simulink model "torqueWalking"  (Simulink 8.9)
settings: Solver=FixedStepAuto  StartTime=0.0  StopTime=CONFIG.SIMULATION_TIME  FixedStep=CONFIG.Ts  RelTol=1e-3
InitFcn:
  | initTorqueWalking
undefined symbols (not defined in the file or in its folder): CONFIG, frictionConeConstraintsMatrix, gain, reg, ROBOT_DOF, root_displacement, upperBoundFrictionConeConstraints, WBT_robotName
undefined symbols (not defined in the file): sat
libraries: WBToolboxLibrary x35
settings Model: SuppressorTable=22 serialization::archive 11 0 6 0 0 0 11 0  Creator=mcharbonneau  LastModifiedBy=mcharbonneau
settings DataIOCC: LimitDataPoints=off  SaveFormat=Dataset  SignalLoggingSaveFormat=Dataset
settings OptimizationCC: LifeSpan=auto
settings DebuggingCC: UnderspecifiedInitializationDetection=Simplified  MergeDetectMultiDrivingBlocksExec=error  FcnCallInpInsideContextMsg=error  StateNameClashWarn=none  SFUnexpectedBacktrackingDiag=error  SFNoUnconditionalDefaultTransitionDiag=error  SFExecutionAtInitializationDiag=warning
settings HardwareCC: ProdBitPerPointer=64  ProdBitPerSizeT=64  ProdBitPerPtrDiffT=64  ProdLargestAtomicFloat=Float  ProdIntDivRoundTo=Zero  ProdEndianess=LittleEndian  ProdWordSize=64  ProdHWDeviceType=Intel->x86-64 (Windows64)
settings ModelReferenceCC: PropagateSignalLabelsOutOfModel=on
settings GRTTargetCC: TargetLangStandard=C99 (ISO)  GeneratePreprocessorConditionals=Use local settings  CombineOutputUpdateFcns=on  GRTInterface=off
settings ConfigComp: CovMetricSettings=dwe  CovHtmlReporting=off  CovSaveCumulativeToWorkspaceVar=off  CovSaveSingleToWorkspaceVar=off  CovExternalEMLEnable=on

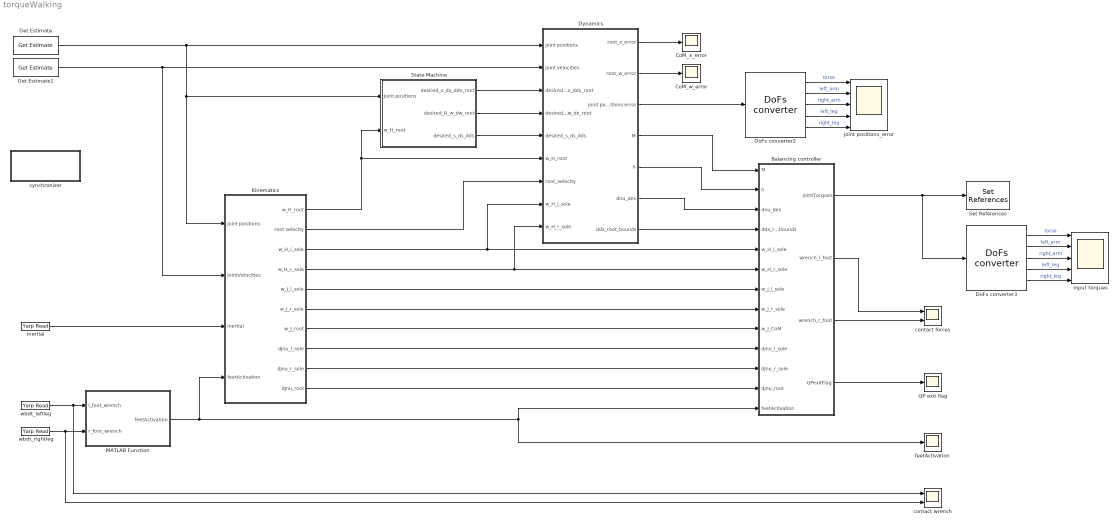
== system torqueWalking ==
  Balancing controller : Subsystem
  CoM_w_error : Scope
  CoM_x_error : Scope
  DoFs converter2 : WBToolboxLibrary/Utilities/DoFs converter  yarp2WBIOption=From WBI to YARP  robotName=WBT_robotName  localName=WBT_modelName  wbiFile=WBT_wbiFilename  wbiList=WBT_wbiList
      settings: SourceProductName=Whole Body Toolbox
  DoFs converter3 : WBToolboxLibrary/Utilities/DoFs converter  yarp2WBIOption=From WBI to YARP  robotName=WBT_robotName  localName=WBT_modelName  wbiFile=WBT_wbiFilename  wbiList=WBT_wbiList
      settings: SourceProductName=Whole Body Toolbox
  Dynamics : Subsystem
  Get Estimate : WBToolboxLibrary/wholeBodyStates/Get Estimate  estimateType=Joints Position  robotName=WBT_robotName  localName=WBT_modelName  wbiFile=WBT_wbiFilename  wbiList=WBT_wbiList
      settings: SourceProductName=Whole Body Toolbox
  Get Estimate1 : WBToolboxLibrary/wholeBodyStates/Get Estimate  estimateType=Joints Velocity  robotName=WBT_robotName  localName=WBT_modelName  wbiFile=WBT_wbiFilename  wbiList=WBT_wbiList
      settings: SourceProductName=Whole Body Toolbox
  Kinematics : Subsystem
  MATLAB Function : MATLAB Function  TreatAsAtomicUnit=on
  QP exit flag : Scope
  Set References : WBToolboxLibrary/wholeBodyActuators/Set References  controlType=Torque  fullOrSubControl=Full  controlledJoints=''  robotName=WBT_robotName  localName=WBT_modelName  wbiFile=WBT_wbiFilename  wbiList=WBT_wbiList
      settings: SourceProductName=Whole Body Toolbox
  State Machine : Subsystem
  contact forces : Scope  NumInputPorts=2
  contact wrench : Scope  NumInputPorts=2
  feetActivation : Scope
  inertial : WBToolboxLibrary/Utilities/Yarp Read  portName=PORTS.IMU  signalSize=12  blocking=off  timestamp=off  autoconnect=on  errorOnConnection=on
      settings: SourceProductName=Whole Body Toolbox
  input torques : Scope  NumInputPorts=5
  joint positions_error : Scope  NumInputPorts=5
  synchronizer : Subsystem
      mask Display: disp('SYNCHRONIZER')
  wbdt_leftleg : WBToolboxLibrary/Utilities/Yarp Read  portName=PORTS.WBDT_LEFTLEG_EE  signalSize=6  blocking=off  timestamp=off  autoconnect=on  errorOnConnection=on
      settings: SourceProductName=Whole Body Toolbox
  wbdt_rightleg : WBToolboxLibrary/Utilities/Yarp Read  portName=PORTS.WBDT_RIGHTLEG_EE  signalSize=6  blocking=off  timestamp=off  autoconnect=on  errorOnConnection=on
      settings: SourceProductName=Whole Body Toolbox
  wires:
  Get Estimate/1 -> Kinematics/1(joint positions), State Machine/1(joint positions), Dynamics/1(joint positions)
  wbdt_leftleg/1 -> contact wrench/1, MATLAB Function/1(l_foot_wrench)
  inertial/1 -> Kinematics/3(inertial)
  wbdt_rightleg/1 -> contact wrench/2, MATLAB Function/2(r_foot_wrench)
  MATLAB Function/1(feetActivation) -> Kinematics/4(feetActivation), Balancing controller/13(feetActivation), feetActivation/1
  Get Estimate1/1 -> Kinematics/2(jointVelocities), Dynamics/2(joint velocities)
  Kinematics/1(w_H_root) -> State Machine/2(w_H_root), Dynamics/6(w_H_root)
  State Machine/1(desired_x_dx_ddx_root) -> Dynamics/3(desired_x_dx_ddx_root)
  State Machine/2(desired_R_w_dw_root) -> Dynamics/4(desired_R_w_dx_root)
  Dynamics/3(joint positions error) -> DoFs converter2/1
  Dynamics/2(root_w_error) -> CoM_w_error/1
  Dynamics/1(root_x_error) -> CoM_x_error/1
  Dynamics/4(M) -> Balancing controller/1(M)
  Dynamics/5(h) -> Balancing controller/2(h)
  Dynamics/6(dnu_des) -> Balancing controller/3(dnu_des)
  Kinematics/3(w_H_l_sole) -> Dynamics/8(w_H_l_sole), Balancing controller/5(w_H_l_sole)
  Kinematics/4(w_H_r_sole) -> Dynamics/9(w_H_r_sole), Balancing controller/6(w_H_r_sole)
  Kinematics/5(w_J_l_sole) -> Balancing controller/7(w_J_l_sole)
  Kinematics/6(w_J_r_sole) -> Balancing controller/8(w_J_r_sole)
  Kinematics/8(dJnu_l_sole) -> Balancing controller/10(dJnu_l_sole)
  Kinematics/9(dJnu_r_sole) -> Balancing controller/11(dJnu_r_sole)
  Balancing controller/2(wrench_l_foot) -> contact forces/1
  Balancing controller/3(wrench_r_foot) -> contact forces/2
  Balancing controller/4(QPexitFlag) -> QP exit flag/1
  Dynamics/7(ddx_root_bounds) -> Balancing controller/4(ddx_root_bounds)
  Kinematics/10(dJnu_root) -> Balancing controller/12(dJnu_root)
  Kinematics/7(w_J_root) -> Balancing controller/9(w_J_CoM)
  DoFs converter2/2 -> joint positions_error/2  "left_arm"
  DoFs converter2/4 -> joint positions_error/4  "left_leg"
  DoFs converter2/3 -> joint positions_error/3  "right_arm"
  DoFs converter2/1 -> joint positions_error/1  "torso"
  DoFs converter2/5 -> joint positions_error/5  "right_leg"
  Balancing controller/1(jointTorques) -> DoFs converter3/1, Set References/1
  DoFs converter3/5 -> input torques/5  "right_leg"
  DoFs converter3/4 -> input torques/4  "left_leg"
  DoFs converter3/2 -> input torques/2  "left_arm"
  DoFs converter3/3 -> input torques/3  "right_arm"
  DoFs converter3/1 -> input torques/1  "torso"
  State Machine/3(desired_s_ds_dds) -> Dynamics/5(desired_s_ds_dds)
  Kinematics/2(root velocity) -> Dynamics/7(root_velocity)

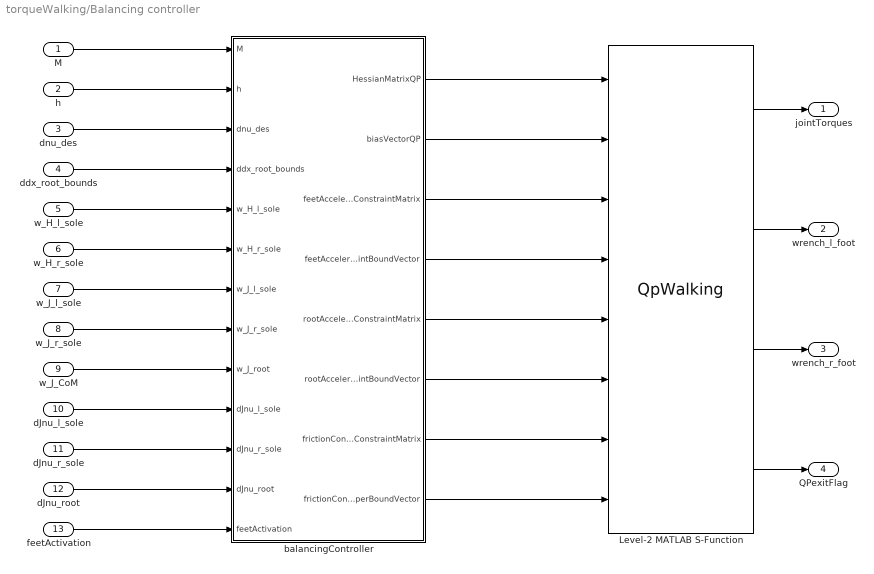
== system torqueWalking/Balancing controller ==
  M : Inport
  h : Inport  Port=2
  dnu_des : Inport  Port=3
  ddx_root_bounds : Inport  Port=4
  w_H_l_sole : Inport  Port=5
  w_H_r_sole : Inport  Port=6
  w_J_l_sole : Inport  Port=7
  w_J_r_sole : Inport  Port=8
  w_J_CoM : Inport  Port=9
  dJnu_l_sole : Inport  Port=10
  dJnu_r_sole : Inport  Port=11
  dJnu_root : Inport  Port=12
  feetActivation : Inport  Port=13
  Level-2 MATLAB S-Function : M-S-Function  FunctionName=QpWalking  Parameters=ROBOT_DOF, constants  mask{robotDofs=ROBOT_DOF, tauDotMax=sat.torqueDot, Ts=CONFIG.Ts}
      mask prompts: robotDofs "Robt degrees of freedom"; tauDotMax "Maximum derivative of torques"; Ts "Controller period"
      mask Display: disp('QP')
  balancingController : MATLAB Function  TreatAsAtomicUnit=on
  jointTorques : Outport
  wrench_l_foot : Outport  Port=2
  wrench_r_foot : Outport  Port=3
  QPexitFlag : Outport  Port=4
  wires:
  feetActivation/1 -> balancingController/13(feetActivation)
  w_J_l_sole/1 -> balancingController/7(w_J_l_sole)
  w_J_r_sole/1 -> balancingController/8(w_J_r_sole)
  M/1 -> balancingController/1(M)
  h/1 -> balancingController/2(h)
  dJnu_l_sole/1 -> balancingController/10(dJnu_l_sole)
  dJnu_r_sole/1 -> balancingController/11(dJnu_r_sole)
  w_H_r_sole/1 -> balancingController/6(w_H_r_sole)
  w_H_l_sole/1 -> balancingController/5(w_H_l_sole)
  balancingController/8(frictionConeUpperBoundVector) -> Level-2 MATLAB S-Function/8
  balancingController/7(frictionConeConstraintMatrix) -> Level-2 MATLAB S-Function/7
  balancingController/4(feetAccelerationConstraintBoundVector) -> Level-2 MATLAB S-Function/4
  balancingController/3(feetAccelerationConstraintMatrix) -> Level-2 MATLAB S-Function/3
  balancingController/2(biasVectorQP) -> Level-2 MATLAB S-Function/2
  balancingController/1(HessianMatrixQP) -> Level-2 MATLAB S-Function/1
  Level-2 MATLAB S-Function/4 -> QPexitFlag/1
  Level-2 MATLAB S-Function/1 -> jointTorques/1
  Level-2 MATLAB S-Function/2 -> wrench_l_foot/1
  Level-2 MATLAB S-Function/3 -> wrench_r_foot/1
  dnu_des/1 -> balancingController/3(dnu_des)
  ddx_root_bounds/1 -> balancingController/4(ddx_root_bounds)
  w_J_CoM/1 -> balancingController/9(w_J_root)
  dJnu_root/1 -> balancingController/12(dJnu_root)
  balancingController/6(rootAccelerationConstraintBoundVector) -> Level-2 MATLAB S-Function/6
  balancingController/5(rootAccelerationConstraintMatrix) -> Level-2 MATLAB S-Function/5

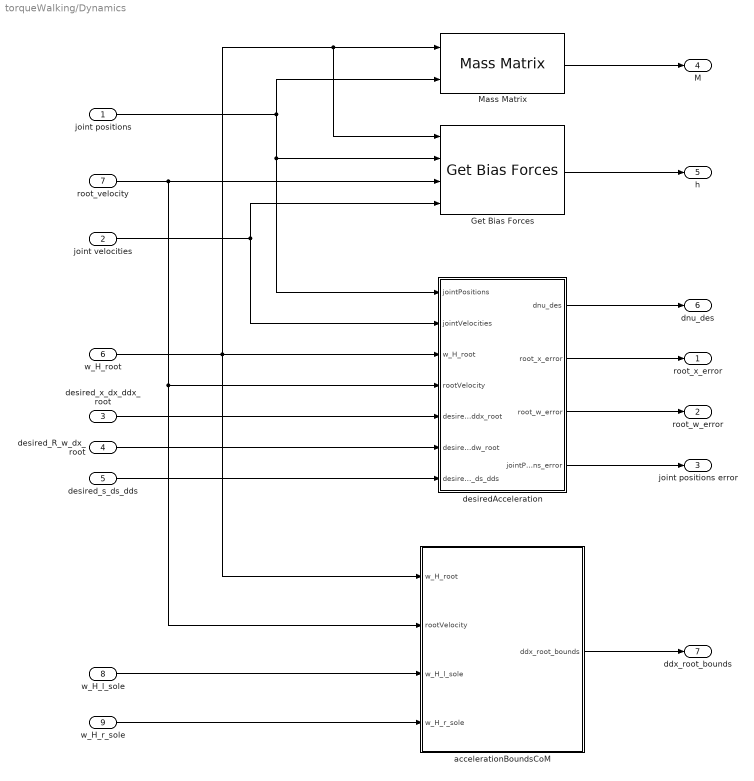
== system torqueWalking/Dynamics ==
  joint positions : Inport
  joint velocities : Inport  Port=2
  desired_x_dx_ddx_root : Inport  Port=3
  desired_R_w_dx_root : Inport  Port=4
  desired_s_ds_dds : Inport  Port=5
  w_H_root : Inport  Port=6
  root_velocity : Inport  Port=7
  w_H_l_sole : Inport  Port=8
  w_H_r_sole : Inport  Port=9
  Get Bias Forces : WBToolboxLibrary/wholeBodyModel/Dynamics/Get Bias Forces  robotName=WBT_robotName  localName=WBT_modelName  wbiFile=WBT_wbiFilename  wbiList=WBT_wbiList  explicitGravity=off
      settings: SourceProductName=Whole Body Toolbox
  Mass Matrix : WBToolboxLibrary/wholeBodyModel/Dynamics/Mass Matrix  robotName=WBT_robotName  localName=WBT_modelName  wbiFile=WBT_wbiFilename  wbiList=WBT_wbiList
      settings: SourceProductName=Whole Body Toolbox
  accelerationBoundsCoM : MATLAB Function  TreatAsAtomicUnit=on
  desiredAcceleration : MATLAB Function  TreatAsAtomicUnit=on
  root_x_error : Outport
  root_w_error : Outport  Port=2
  joint positions error : Outport  Port=3
  M : Outport  Port=4
  h : Outport  Port=5
  dnu_des : Outport  Port=6
  ddx_root_bounds : Outport  Port=7
  wires:
  Mass Matrix/1 -> M/1
  joint velocities/1 -> Get Bias Forces/4, desiredAcceleration/2(jointVelocities)
  w_H_root/1 -> Get Bias Forces/1, Mass Matrix/1, accelerationBoundsCoM/1(w_H_root), desiredAcceleration/3(w_H_root)
  Get Bias Forces/1 -> h/1
  joint positions/1 -> Mass Matrix/2, desiredAcceleration/1(jointPositions), Get Bias Forces/2
  root_velocity/1 -> accelerationBoundsCoM/2(rootVelocity), desiredAcceleration/4(rootVelocity), Get Bias Forces/3
  desiredAcceleration/1(dnu_des) -> dnu_des/1
  desired_x_dx_ddx_root/1 -> desiredAcceleration/5(desired_x_dx_ddx_root)
  desired_R_w_dx_root/1 -> desiredAcceleration/6(desired_R_w_dw_root)
  desired_s_ds_dds/1 -> desiredAcceleration/7(desired_s_ds_dds)
  desiredAcceleration/2(root_x_error) -> root_x_error/1
  desiredAcceleration/3(root_w_error) -> root_w_error/1
  desiredAcceleration/4(jointPositions_error) -> joint positions error/1
  w_H_l_sole/1 -> accelerationBoundsCoM/3(w_H_l_sole)
  w_H_r_sole/1 -> accelerationBoundsCoM/4(w_H_r_sole)
  accelerationBoundsCoM/1(ddx_root_bounds) -> ddx_root_bounds/1

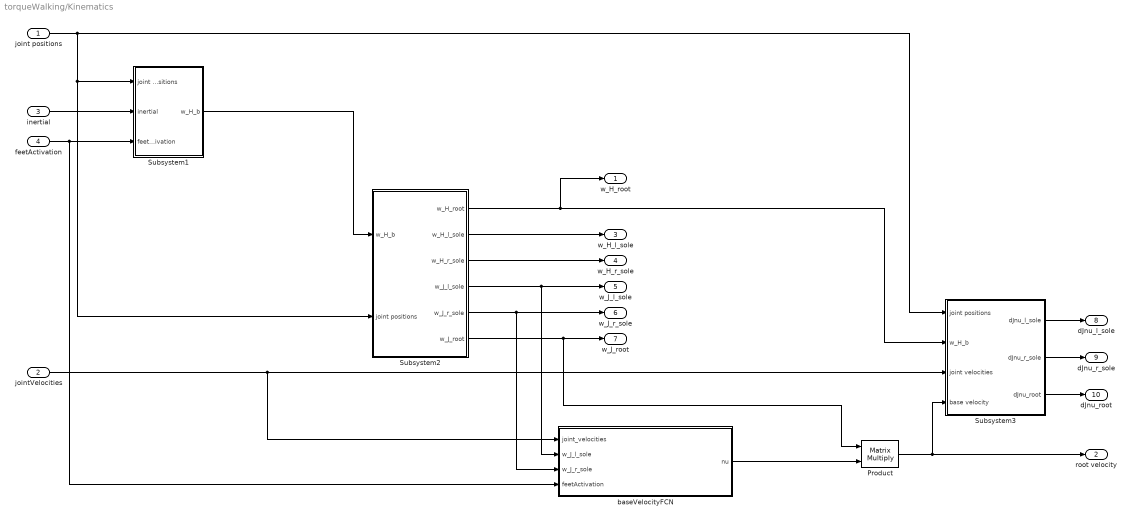
== system torqueWalking/Kinematics ==
  joint positions : Inport
  jointVelocities : Inport  Port=2
  inertial : Inport  Port=3
  feetActivation : Inport  Port=4
  Product : Product  Multiplication=Matrix(*)
  Subsystem1 : Subsystem
  Subsystem2 : Subsystem
  Subsystem3 : Subsystem
  baseVelocityFCN : MATLAB Function  TreatAsAtomicUnit=on
  w_H_root : Outport
  root velocity : Outport  Port=2
  w_H_l_sole : Outport  Port=3
  w_H_r_sole : Outport  Port=4
  w_J_l_sole : Outport  Port=5
  w_J_r_sole : Outport  Port=6
  w_J_root : Outport  Port=7
  dJnu_l_sole : Outport  Port=8
  dJnu_r_sole : Outport  Port=9
  dJnu_root : Outport  Port=10
  wires:
  inertial/1 -> Subsystem1/2(inertial)
  joint positions/1 -> Subsystem2/2(joint positions), Subsystem1/1(joint positions), Subsystem3/1(joint positions)
  feetActivation/1 -> baseVelocityFCN/4(feetActivation), Subsystem1/3(feetActivation)
  Subsystem1/1(w_H_b) -> Subsystem2/1(w_H_b)
  Subsystem2/4(w_J_l_sole) -> w_J_l_sole/1, baseVelocityFCN/2(w_J_l_sole)
  Subsystem2/5(w_J_r_sole) -> w_J_r_sole/1, baseVelocityFCN/3(w_J_r_sole)
  jointVelocities/1 -> baseVelocityFCN/1(joint_velocities), Subsystem3/3(joint velocities)
  Subsystem3/1(dJnu_l_sole) -> dJnu_l_sole/1
  Subsystem3/2(dJnu_r_sole) -> dJnu_r_sole/1
  Subsystem2/1(w_H_root) -> w_H_root/1, Subsystem3/2(w_H_b)
  Subsystem2/6(w_J_root) -> w_J_root/1, Product/1
  baseVelocityFCN/1(nu) -> Product/2
  Product/1 -> root velocity/1, Subsystem3/4(base velocity)
  Subsystem2/2(w_H_l_sole) -> w_H_l_sole/1
  Subsystem2/3(w_H_r_sole) -> w_H_r_sole/1
  Subsystem3/3(dJnu_root) -> dJnu_root/1

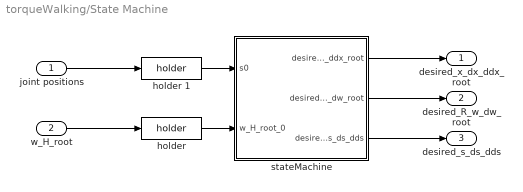
== system torqueWalking/State Machine ==
  joint positions : Inport
  w_H_root : Inport  Port=2
  "holder " : WBToolboxLibrary/Utilities/holder 
      settings: SourceProductName=Whole Body Toolbox
  holder 1 : WBToolboxLibrary/Utilities/holder 
      settings: SourceProductName=Whole Body Toolbox
  stateMachine : MATLAB Function  TreatAsAtomicUnit=on
  desired_x_dx_ddx_root : Outport
  desired_R_w_dw_root : Outport  Port=2
  desired_s_ds_dds : Outport  Port=3
  wires:
  stateMachine/2(desired_R_w_dw_root) -> desired_R_w_dw_root/1
  stateMachine/3(desired_s_ds_dds) -> desired_s_ds_dds/1
  holder 1/1 -> stateMachine/1(s0)
  w_H_root/1 -> "holder "/1
  joint positions/1 -> holder 1/1
  "holder "/1 -> stateMachine/2(w_H_root_0)
  stateMachine/1(desired_x_dx_ddx_root) -> desired_x_dx_ddx_root/1

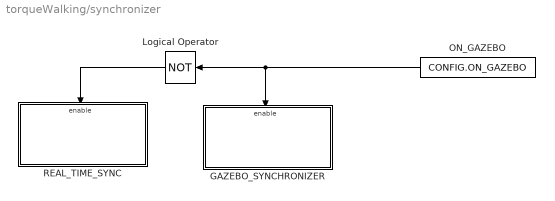
== system torqueWalking/synchronizer ==
  GAZEBO_SYNCHRONIZER : Subsystem
  Logical Operator : Logic  Operator=NOT  AllPortsSameDT=off  OutDataTypeStr=boolean
  "ON_GAZEBO " : Constant  Value=CONFIG.ON_GAZEBO
  REAL_TIME_SYNC : Subsystem
  wires:
  Logical Operator/1 -> REAL_TIME_SYNC/Enable
  "ON_GAZEBO "/1 -> GAZEBO_SYNCHRONIZER/Enable, Logical Operator/1

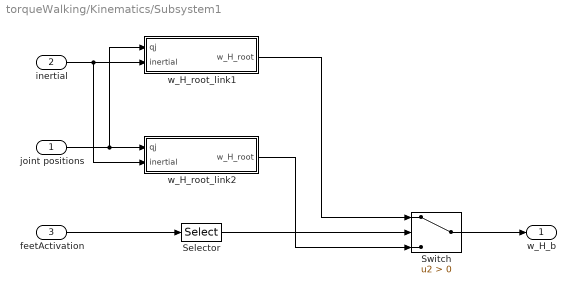
== system torqueWalking/Kinematics/Subsystem1 ==
  joint positions : Inport
  inertial : Inport  Port=2
  feetActivation : Inport  Port=3
  Selector : Selector  InputPortWidth=2  IndexOptions=Index vector (dialog)  Indices=[1]  OutputSizes=1
  Switch : Switch  Criteria=u2 > Threshold
  w_H_root_link1 : Subsystem  mask{link_name='l_sole'}
      mask prompts: link_name "link name"
      mask help:
      | This block evaluates the homogeneous transformation between the world and the root link, i.e. ^wH_b. It assumes that the link specified by the variable 'link_name' has a constant position
      | w.r.t. an inertial frame, but it can rotate arbitrarily. This rotation is retrived from the IMU sensor.
      mask Display:
      | str = strrep(link_name, '_','\_');
      | port_label('output',1,['{}^{',str '}H_{root}'],'texmode','on')
      | clear str;
      | 
      | port_label('input',1,'q_j','texmode','on')
      | 
      | port_label('input',2,'inertial','texmode','on')
  w_H_root_link2 : Subsystem  mask{link_name='r_sole'}
      mask prompts: link_name "link name"
      mask help:
      | This block evaluates the homogeneous transformation between the world and the root link, i.e. ^wH_b. It assumes that the link specified by the variable 'link_name' has a constant position
      | w.r.t. an inertial frame, but it can rotate arbitrarily. This rotation is retrived from the IMU sensor.
      mask Display:
      | str = strrep(link_name, '_','\_');
      | port_label('output',1,['{}^{',str '}H_{root}'],'texmode','on')
      | clear str;
      | 
      | port_label('input',1,'q_j','texmode','on')
      | 
      | port_label('input',2,'inertial','texmode','on')
  w_H_b : Outport
  wires:
  w_H_root_link1/1(w_H_root) -> Switch/1
  joint positions/1 -> w_H_root_link2/1(qj), w_H_root_link1/1(qj)
  inertial/1 -> w_H_root_link2/2(inertial), w_H_root_link1/2(inertial)
  w_H_root_link2/1(w_H_root) -> Switch/3
  feetActivation/1 -> Selector/1
  Selector/1 -> Switch/2
  Switch/1 -> w_H_b/1

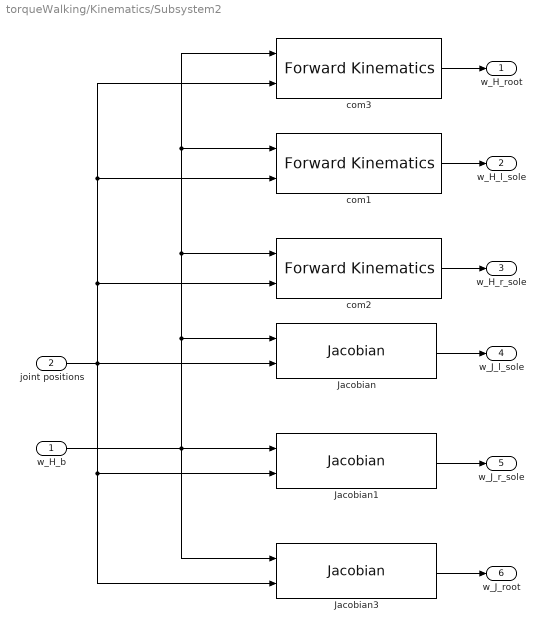
== system torqueWalking/Kinematics/Subsystem2 ==
  w_H_b : Inport
  joint positions : Inport  Port=2
  Jacobian : WBToolboxLibrary/wholeBodyModel/Jacobians/Jacobian  frameName='l_sole'  robotName=WBT_robotName  localName=WBT_modelName  wbiFile=WBT_wbiFilename  wbiList=WBT_wbiList
      settings: SourceProductName=Whole Body Toolbox
  Jacobian1 : WBToolboxLibrary/wholeBodyModel/Jacobians/Jacobian  frameName='r_sole'  robotName=WBT_robotName  localName=WBT_modelName  wbiFile=WBT_wbiFilename  wbiList=WBT_wbiList
      settings: SourceProductName=Whole Body Toolbox
  Jacobian3 : WBToolboxLibrary/wholeBodyModel/Jacobians/Jacobian  frameName=FRAMES.BASE  robotName=WBT_robotName  localName=WBT_modelName  wbiFile=WBT_wbiFilename  wbiList=WBT_wbiList
      settings: SourceProductName=Whole Body Toolbox
  com1 : WBToolboxLibrary/wholeBodyModel/Kinematics/Forward Kinematics  frameName='l_sole'  robotName=WBT_robotName  localName=WBT_modelName  wbiFile=WBT_wbiFilename  wbiList=WBT_wbiList
      settings: SourceProductName=Whole Body Toolbox
  com2 : WBToolboxLibrary/wholeBodyModel/Kinematics/Forward Kinematics  frameName='r_sole'  robotName=WBT_robotName  localName=WBT_modelName  wbiFile=WBT_wbiFilename  wbiList=WBT_wbiList
      settings: SourceProductName=Whole Body Toolbox
  com3 : WBToolboxLibrary/wholeBodyModel/Kinematics/Forward Kinematics  frameName=FRAMES.BASE  robotName=WBT_robotName  localName=WBT_modelName  wbiFile=WBT_wbiFilename  wbiList=WBT_wbiList
      settings: SourceProductName=Whole Body Toolbox
  w_H_root : Outport
  w_H_l_sole : Outport  Port=2
  w_H_r_sole : Outport  Port=3
  w_J_l_sole : Outport  Port=4
  w_J_r_sole : Outport  Port=5
  w_J_root : Outport  Port=6
  wires:
  Jacobian/1 -> w_J_l_sole/1
  w_H_b/1 -> com2/1, com3/1, com1/1, Jacobian/1, Jacobian3/1, Jacobian1/1
  joint positions/1 -> com2/2, com1/2, com3/2, Jacobian3/2, Jacobian1/2, Jacobian/2
  Jacobian1/1 -> w_J_r_sole/1
  com1/1 -> w_H_l_sole/1
  com2/1 -> w_H_r_sole/1
  Jacobian3/1 -> w_J_root/1
  com3/1 -> w_H_root/1

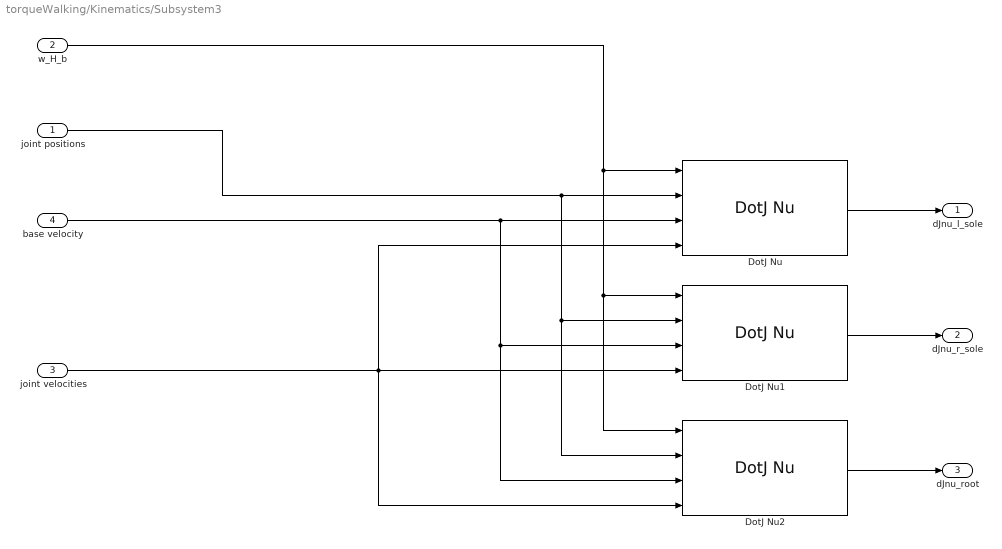
== system torqueWalking/Kinematics/Subsystem3 ==
  joint positions : Inport
  w_H_b : Inport  Port=2
  joint velocities : Inport  Port=3
  base velocity : Inport  Port=4
  DotJ Nu : WBToolboxLibrary/wholeBodyModel/Jacobians/DotJ Nu  frameName='l_sole'  robotName=WBT_robotName  localName=WBT_modelName  wbiFile=WBT_wbiFilename  wbiList=WBT_wbiList
      settings: SourceProductName=Whole Body Toolbox
  DotJ Nu1 : WBToolboxLibrary/wholeBodyModel/Jacobians/DotJ Nu  frameName='l_sole'  robotName=WBT_robotName  localName=WBT_modelName  wbiFile=WBT_wbiFilename  wbiList=WBT_wbiList
      settings: SourceProductName=Whole Body Toolbox
  DotJ Nu2 : WBToolboxLibrary/wholeBodyModel/Jacobians/DotJ Nu  frameName=FRAMES.BASE  robotName=WBT_robotName  localName=WBT_modelName  wbiFile=WBT_wbiFilename  wbiList=WBT_wbiList
      settings: SourceProductName=Whole Body Toolbox
  dJnu_l_sole : Outport
  dJnu_r_sole : Outport  Port=2
  dJnu_root : Outport  Port=3
  wires:
  base velocity/1 -> DotJ Nu2/3, DotJ Nu1/3, DotJ Nu/3
  joint velocities/1 -> DotJ Nu2/4, DotJ Nu1/4, DotJ Nu/4
  DotJ Nu1/1 -> dJnu_r_sole/1
  joint positions/1 -> DotJ Nu2/2, DotJ Nu1/2, DotJ Nu/2
  DotJ Nu/1 -> dJnu_l_sole/1
  w_H_b/1 -> DotJ Nu/1, DotJ Nu1/1, DotJ Nu2/1
  DotJ Nu2/1 -> dJnu_root/1

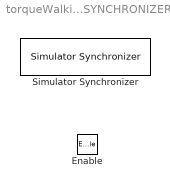
== system torqueWalking/synchronizer/GAZEBO_SYNCHRONIZER ==
  Enable : EnablePort
  Simulator Synchronizer : WBToolboxLibrary/Utilities/Simulator Synchronizer  period=CONFIG.Ts  serverPortName='/clock/rpc'  clientPortName='/WBT_synchronizer/rpc:o'
      settings: SourceProductName=Whole Body Toolbox

== system torqueWalking/synchronizer/REAL_TIME_SYNC ==
  Enable : EnablePort
  Real Time Synchronizer : WBToolboxLibrary/Utilities/Real Time Synchronizer  period=CONFIG.Ts
      settings: SourceProductName=Whole Body Toolbox

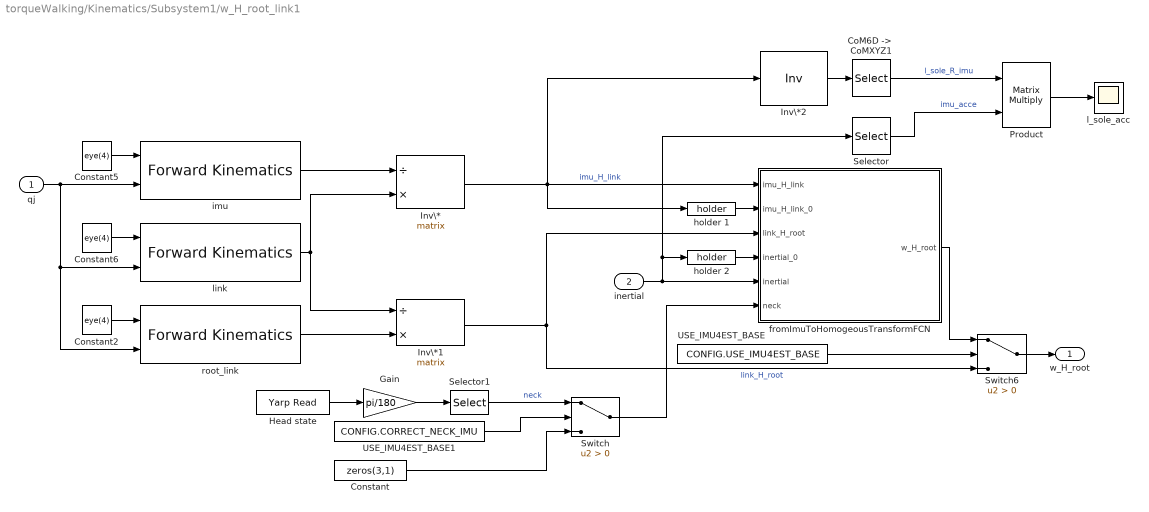
== system torqueWalking/Kinematics/Subsystem1/w_H_root_link1 ==
  qj : Inport
  inertial : Inport  Port=2
  "CoM6D ->  CoMXYZ1" : Selector  NumberOfDimensions=2  InputPortWidth=7  IndexOptions=Index vector (dialog),Index vector (dialog)  Indices=[1 2 3],[1 2 3]  OutputSizes=1,1
  Constant : Constant  Value=zeros(3,1)
  Constant2 : Constant  Value=eye(4)
  Constant5 : Constant  Value=eye(4)
  Constant6 : Constant  Value=eye(4)
  Gain : Gain  Gain=pi/180
  Head state : WBToolboxLibrary/Utilities/Yarp Read  portName=[WBT_robotName, '/head/state:o']  signalSize=6  blocking=off  timestamp=off  autoconnect=on  errorOnConnection=off
      settings: SourceProductName=Whole Body Toolbox
  Inv\* : Product  Inputs=/*  Multiplication=Matrix(*)
  Inv\*1 : Product  Inputs=/*  Multiplication=Matrix(*)
  Inv\*2 : Product  Inputs=/  Multiplication=Matrix(*)
  Product : Product  Multiplication=Matrix(*)
  Selector : Selector  InputPortWidth=12  IndexOptions=Index vector (dialog)  Indices=[4 5 6 ]  OutputSizes=1
  Selector1 : Selector  InputPortWidth=6  IndexOptions=Index vector (dialog)  Indices=[1:3]  OutputSizes=1
  Switch : Switch  Criteria=u2 > Threshold
  Switch6 : Switch  Criteria=u2 > Threshold
  USE_IMU4EST_BASE : Constant  Value=CONFIG.USE_IMU4EST_BASE
  USE_IMU4EST_BASE1 : Constant  Value=CONFIG.CORRECT_NECK_IMU
  fromImuToHomogeousTransformFCN : MATLAB Function  TreatAsAtomicUnit=on
  holder 1 : WBToolboxLibrary/Utilities/holder 
      settings: SourceProductName=Whole Body Toolbox
  holder 2 : WBToolboxLibrary/Utilities/holder 
      settings: SourceProductName=Whole Body Toolbox
  imu : WBToolboxLibrary/wholeBodyModel/Kinematics/Forward Kinematics  frameName='imu_frame'  robotName=WBT_robotName  localName=WBT_modelName  wbiFile=WBT_wbiFilename  wbiList=WBT_wbiList
      settings: SourceProductName=Whole Body Toolbox
  l_sole_acc : Scope
  link : WBToolboxLibrary/wholeBodyModel/Kinematics/Forward Kinematics  frameName=link_name  robotName=WBT_robotName  localName=WBT_modelName  wbiFile=WBT_wbiFilename  wbiList=WBT_wbiList
      settings: SourceProductName=Whole Body Toolbox
  root_link : WBToolboxLibrary/wholeBodyModel/Kinematics/Forward Kinematics  frameName=FRAMES.BASE  robotName=WBT_robotName  localName=WBT_modelName  wbiFile=WBT_wbiFilename  wbiList=WBT_wbiList
      settings: SourceProductName=Whole Body Toolbox
  w_H_root : Outport
  wires:
  Constant/1 -> Switch/3
  Gain/1 -> Selector1/1
  Switch/1 -> fromImuToHomogeousTransformFCN/6(neck)
  USE_IMU4EST_BASE1/1 -> Switch/2
  Selector1/1 -> Switch/1  "neck"
  Head state/1 -> Gain/1
  Product/1 -> l_sole_acc/1
  Selector/1 -> Product/2  "imu_acce"
  "CoM6D ->  CoMXYZ1"/1 -> Product/1  "l_sole_R_imu"
  Inv\*2/1 -> "CoM6D ->  CoMXYZ1"/1
  holder 2/1 -> fromImuToHomogeousTransformFCN/4(inertial_0)
  holder 1/1 -> fromImuToHomogeousTransformFCN/2(imu_H_link_0)
  root_link/1 -> Inv\*1/2
  qj/1 -> imu/2, link/2, root_link/2
  Constant2/1 -> root_link/1
  fromImuToHomogeousTransformFCN/1(w_H_root) -> Switch6/1
  USE_IMU4EST_BASE/1 -> Switch6/2
  Switch6/1 -> w_H_root/1
  inertial/1 -> fromImuToHomogeousTransformFCN/5(inertial), holder 2/1, Selector/1
  link/1 -> Inv\*1/1, Inv\*/2
  Inv\*1/1 -> fromImuToHomogeousTransformFCN/3(link_H_root), Switch6/3  "link_H_root"
  Constant6/1 -> link/1
  imu/1 -> Inv\*/1
  Inv\*/1 -> fromImuToHomogeousTransformFCN/1(imu_H_link), holder 1/1, Inv\*2/1  "imu_H_link"
  Constant5/1 -> imu/1

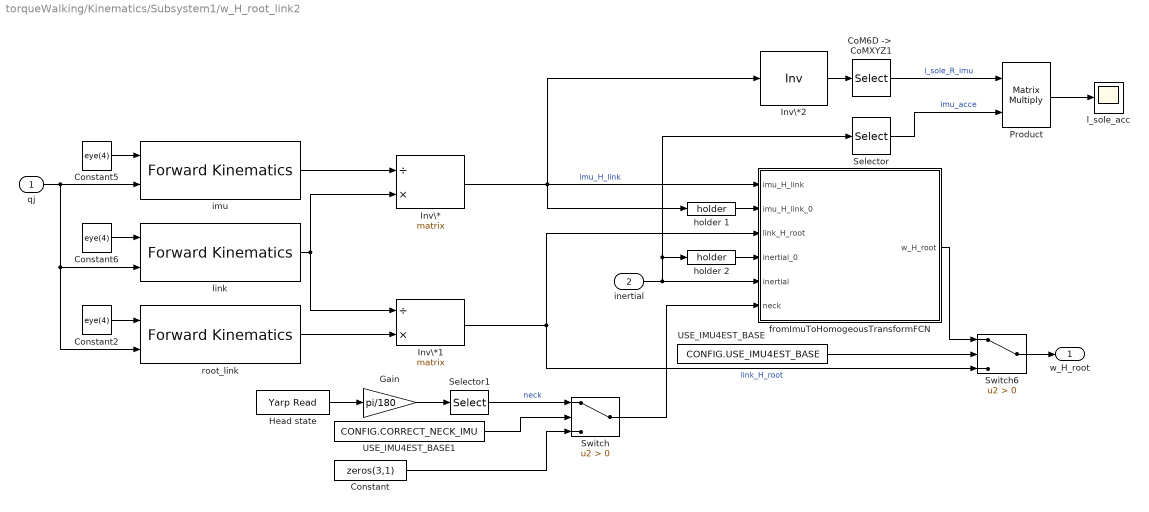
== system torqueWalking/Kinematics/Subsystem1/w_H_root_link2 ==
  qj : Inport
  inertial : Inport  Port=2
  "CoM6D ->  CoMXYZ1" : Selector  NumberOfDimensions=2  InputPortWidth=7  IndexOptions=Index vector (dialog),Index vector (dialog)  Indices=[1 2 3],[1 2 3]  OutputSizes=1,1
  Constant : Constant  Value=zeros(3,1)
  Constant2 : Constant  Value=eye(4)
  Constant5 : Constant  Value=eye(4)
  Constant6 : Constant  Value=eye(4)
  Gain : Gain  Gain=pi/180
  Head state : WBToolboxLibrary/Utilities/Yarp Read  portName=[WBT_robotName, '/head/state:o']  signalSize=6  blocking=off  timestamp=off  autoconnect=on  errorOnConnection=off
      settings: SourceProductName=Whole Body Toolbox
  Inv\* : Product  Inputs=/*  Multiplication=Matrix(*)
  Inv\*1 : Product  Inputs=/*  Multiplication=Matrix(*)
  Inv\*2 : Product  Inputs=/  Multiplication=Matrix(*)
  Product : Product  Multiplication=Matrix(*)
  Selector : Selector  InputPortWidth=12  IndexOptions=Index vector (dialog)  Indices=[4 5 6 ]  OutputSizes=1
  Selector1 : Selector  InputPortWidth=6  IndexOptions=Index vector (dialog)  Indices=[1:3]  OutputSizes=1
  Switch : Switch  Criteria=u2 > Threshold
  Switch6 : Switch  Criteria=u2 > Threshold
  USE_IMU4EST_BASE : Constant  Value=CONFIG.USE_IMU4EST_BASE
  USE_IMU4EST_BASE1 : Constant  Value=CONFIG.CORRECT_NECK_IMU
  fromImuToHomogeousTransformFCN : MATLAB Function  TreatAsAtomicUnit=on
  holder 1 : WBToolboxLibrary/Utilities/holder 
      settings: SourceProductName=Whole Body Toolbox
  holder 2 : WBToolboxLibrary/Utilities/holder 
      settings: SourceProductName=Whole Body Toolbox
  imu : WBToolboxLibrary/wholeBodyModel/Kinematics/Forward Kinematics  frameName='imu_frame'  robotName=WBT_robotName  localName=WBT_modelName  wbiFile=WBT_wbiFilename  wbiList=WBT_wbiList
      settings: SourceProductName=Whole Body Toolbox
  l_sole_acc : Scope
  link : WBToolboxLibrary/wholeBodyModel/Kinematics/Forward Kinematics  frameName=link_name  robotName=WBT_robotName  localName=WBT_modelName  wbiFile=WBT_wbiFilename  wbiList=WBT_wbiList
      settings: SourceProductName=Whole Body Toolbox
  root_link : WBToolboxLibrary/wholeBodyModel/Kinematics/Forward Kinematics  frameName=FRAMES.BASE  robotName=WBT_robotName  localName=WBT_modelName  wbiFile=WBT_wbiFilename  wbiList=WBT_wbiList
      settings: SourceProductName=Whole Body Toolbox
  w_H_root : Outport
  wires:
  Constant5/1 -> imu/1
  Inv\*/1 -> Inv\*2/1, holder 1/1, fromImuToHomogeousTransformFCN/1(imu_H_link)  "imu_H_link"
  imu/1 -> Inv\*/1
  Constant6/1 -> link/1
  Inv\*1/1 -> Switch6/3, fromImuToHomogeousTransformFCN/3(link_H_root)  "link_H_root"
  link/1 -> Inv\*/2, Inv\*1/1
  inertial/1 -> Selector/1, holder 2/1, fromImuToHomogeousTransformFCN/5(inertial)
  Switch6/1 -> w_H_root/1
  USE_IMU4EST_BASE/1 -> Switch6/2
  fromImuToHomogeousTransformFCN/1(w_H_root) -> Switch6/1
  Constant2/1 -> root_link/1
  qj/1 -> root_link/2, link/2, imu/2
  root_link/1 -> Inv\*1/2
  holder 1/1 -> fromImuToHomogeousTransformFCN/2(imu_H_link_0)
  holder 2/1 -> fromImuToHomogeousTransformFCN/4(inertial_0)
  Inv\*2/1 -> "CoM6D ->  CoMXYZ1"/1
  "CoM6D ->  CoMXYZ1"/1 -> Product/1  "l_sole_R_imu"
  Selector/1 -> Product/2  "imu_acce"
  Product/1 -> l_sole_acc/1
  Head state/1 -> Gain/1
  Selector1/1 -> Switch/1  "neck"
  USE_IMU4EST_BASE1/1 -> Switch/2
  Switch/1 -> fromImuToHomogeousTransformFCN/6(neck)
  Gain/1 -> Selector1/1
  Constant/1 -> Switch/3

== matlab function Kinematics/Subsystem1/w_H_root_link1/fromImuToHomogeousTransformFCN ==
  data: imu_H_link input double; imu_H_link_0 input double; link_H_root input double; inertial_0 input double; inertial input double; neck input double; w_H_root output double; CONFIG parameter double
function w_H_root = fromBaseToWorldWithImuFCN(imu_H_link,imu_H_link_0,link_H_root,inertial_0,inertial,neck,CONFIG)
%#codegen
w_H_root = fromBaseToWorldWithImu(imu_H_link,imu_H_link_0,link_H_root,inertial_0,inertial,neck,CONFIG);

== matlab function MATLAB Function ==
  data: l_foot_wrench input double; feetActivation output double; r_foot_wrench input double; sm parameter double
function feetActivation = feetActivationFCN(l_foot_wrench, r_foot_wrench, sm)

feetActivation = ones(2,1);

if (l_foot_wrench(3) < sm.wrench.thresholdContactOn)
    feetActivation(1) = 0;
elseif (r_foot_wrench(3) < sm.wrench.thresholdContactOn)
    feetActivation(2) = 0;
end

== matlab function Kinematics/Subsystem1/w_H_root_link2/fromImuToHomogeousTransformFCN ==
  data: imu_H_link input double; imu_H_link_0 input double; link_H_root input double; inertial_0 input double; inertial input double; neck input double; w_H_root output double; CONFIG parameter double
function w_H_root = fromBaseToWorldWithImuFCN(imu_H_link,imu_H_link_0,link_H_root,inertial_0,inertial,neck,CONFIG)
%#codegen
w_H_root = fromBaseToWorldWithImu(imu_H_link,imu_H_link_0,link_H_root,inertial_0,inertial,neck,CONFIG);

== matlab function Balancing controller/balancingController ==
  data: M input double; h input double; dnu_des input double; ddx_root_bounds input double; HessianMatrixQP output double; w_H_l_sole input double; w_H_r_sole input double; w_J_l_sole input double; w_J_r_sole input double; w_J_root input double; dJnu_l_sole input double; dJnu_r_sole input double; dJnu_root input double; feetActivation input double; frictionConeConstraintsMatrix parameter double; upperBoundFrictionConeConstraints parameter double; ROBOT_DOF parameter double; gain parameter double; biasVectorQP output double; feetAccelerationConstraintMatrix output double; feetAccelerationConstraintBoundVector output double; rootAccelerationConstraintMatrix output double; rootAccelerationConstraintBoundVector output double; frictionConeConstraintMatrix output double; frictionConeUpperBoundVector output double; reg parameter double
function [HessianMatrixQP, biasVectorQP, ...
          feetAccelerationConstraintMatrix, feetAccelerationConstraintBoundVector, ...
          rootAccelerationConstraintMatrix, rootAccelerationConstraintBoundVector, ...
          frictionConeConstraintMatrix, frictionConeUpperBoundVector] ...
         = balancingControllerFCN( M, h, dnu_des, ddx_root_bounds, ...
                                w_H_l_sole, w_H_r_sole, w_J_l_sole, w_J_r_sole, w_J_root, ...
                                dJnu_l_sole, dJnu_r_sole, dJnu_root, feetActivation, ...
                                frictionConeConstraintsMatrix, upperBoundFrictionConeConstraints, ...
                                ROBOT_DOF, gain, reg)

                            
[HessianMatrixQP, biasVectorQP, ...
          feetAccelerationConstraintMatrix, feetAccelerationConstraintBoundVector, ...
          rootAccelerationConstraintMatrix, rootAccelerationConstraintBoundVector, ...
          frictionConeConstraintMatrix, frictionConeUpperBoundVector] ...
         = balancingController( M, h, dnu_des, ddx_root_bounds, ...
                                w_H_l_sole, w_H_r_sole, w_J_l_sole, w_J_r_sole, w_J_root, ...
                                dJnu_l_sole, dJnu_r_sole, dJnu_root, feetActivation, ...
                                frictionConeConstraintsMatrix, upperBoundFrictionConeConstraints, ...
                                ROBOT_DOF, gain, reg);

== matlab function Kinematics/baseVelocityFCN ==
  data: joint_velocities input double; w_J_l_sole input double; w_J_r_sole input double; feetActivation input double; reg parameter double; nu output double
function nu  = baseVelocityFCN(joint_velocities, w_J_l_sole, w_J_r_sole, feetActivation, reg)

    nu  = baseVelocity(joint_velocities, w_J_l_sole, w_J_r_sole, feetActivation, reg);

== matlab function Dynamics/desiredAcceleration ==
  data: jointPositions input double; jointVelocities input double; w_H_root input double; rootVelocity input double; desired_x_dx_ddx_root input double; desired_R_w_dw_root input double; desired_s_ds_dds input double; dnu_des output double; gain parameter double; root_x_error output double; root_w_error output double; jointPositions_error output double
function [dnu_des, root_x_error, root_w_error, jointPositions_error] = desiredAcceleration(jointPositions, jointVelocities, w_H_root, rootVelocity, ...
                           desired_x_dx_ddx_root, desired_R_w_dw_root, desired_s_ds_dds, ...
                           gain)
[dnu_des, root_x_error, root_w_error, jointPositions_error] = desiredAcceleration(jointPositions, jointVelocities, w_H_root, rootVelocity, ...
                           desired_x_dx_ddx_root, desired_R_w_dw_root, desired_s_ds_dds, ...
                           gain);

== matlab function State Machine/stateMachine ==
  data: s0 input double; w_H_root_0 input double; desired_x_dx_ddx_root output double; desired_R_w_dw_root output double; desired_s_ds_dds output double; ROBOT_DOF parameter double; root_displacement parameter double
function [desired_x_dx_ddx_root, desired_R_w_dw_root, desired_s_ds_dds] = stateMachine(s0, w_H_root_0, ROBOT_DOF, root_displacement)

[desired_x_dx_ddx_root, desired_R_w_dw_root, desired_s_ds_dds] = stateMachine(s0, w_H_root_0, root_displacement, ROBOT_DOF);

== matlab function Dynamics/accelerationBoundsCoM ==
  data: w_H_root input double; rootVelocity input double; w_H_l_sole input double; w_H_r_sole input double; ddx_root_bounds output double; gain parameter double
function ddx_root_bounds  = CoMaccelerationBoundsFCN(w_H_root, rootVelocity, ...
                           w_H_l_sole, w_H_r_sole, ...
                           gain)

ddx_root_bounds = CoMaccelerationBounds( w_H_root, rootVelocity, ...
                           w_H_l_sole, w_H_r_sole, ...
                           gain );
